simulink model "verify_Cooling_Tower_mdl"  (R2018b)
settings: Solver=ode45  StartTime=0  StopTime=1200  MaxStep=60  RelTol=1e-3  EnableMultiTasking=on
libraries: carnot x3
settings Model: Creator=drhf  LastModifiedBy=drhf
settings DataIOCC: SaveFormat=Array  SignalLoggingSaveFormat=ModelDataLogs
settings OptimizationCC: ExpressionDepthLimit=2147483647  LifeSpan=inf
settings DebuggingCC: UnderspecifiedInitializationDetection=Classic  MergeDetectMultiDrivingBlocksExec=none  SolverPrmCheckMsg=warning  FcnCallInpInsideContextMsg=warning  StateNameClashWarn=warning  SFUnexpectedBacktrackingDiag=warning  SFNoUnconditionalDefaultTransitionDiag=warning  SFExecutionAtInitializationDiag=none
settings HardwareCC: ProdBitPerPointer=32  ProdBitPerSizeT=32  ProdBitPerPtrDiffT=32  ProdLargestAtomicFloat=None  ProdIntDivRoundTo=Undefined  ProdEndianess=Unspecified  ProdWordSize=32  ProdHWDeviceType=32-bit Generic
settings ModelReferenceCC: PropagateSignalLabelsOutOfModel=off
settings SFSimCC: SimUseLocalCustomCode=off
settings RTWCC: RTWUseLocalCustomCode=off
settings CodeAppCC: StateflowObjectComments=on
settings GRTTargetCC: TargetLangStandard=C89/C90 (ANSI)  GeneratePreprocessorConditionals=Disable all  CombineOutputUpdateFcns=off  GRTInterface=on
settings ConfigComp: CovMetricSettings=dw  CovHtmlReporting=on  CovSaveCumulativeToWorkspaceVar=on  CovSaveSingleToWorkspaceVar=on  CovExternalEMLEnable=off

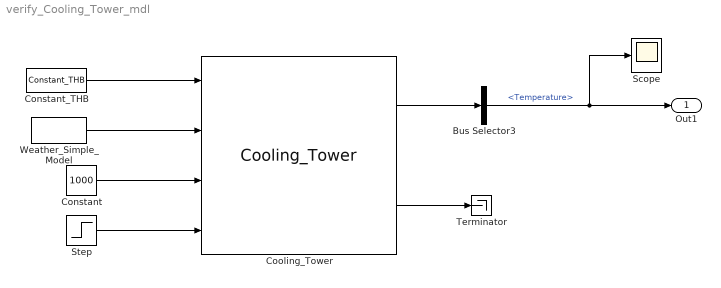
== system verify_Cooling_Tower_mdl ==
  Bus Selector3 : BusSelector  OutputSignals=Temperature
  Constant : Constant  Value=1000
  Constant_THB : carnot/Source/Simple/Constant_THB  t=15  mdot=1200/3600  p=1e5  mID=No Pressure Drop  fluid=Water  mix=0  mix2=0  mix3=0  dia=0.02  hgt=0
      settings: SourceProductName=Carnot
  Cooling_Tower : carnot/Source/Chiller/Cooling_Tower
      settings: SourceProductName=Carnot
  Scope : Scope
  Step : Step  Time=200  SampleTime=0
  Terminator : Terminator
  Weather_Simple_Model : carnot/Weather/Weather_Simple_Model  Ibn=900  Idg=100  tamb=5  deltaTsky=-6  rh=50  precip="10e-3/24/3600           % 10 mm in 24 h"  cloud=0.125  p=1013e2  vw=1  wdir=270  lat=60  colangle=0  colazi=0  colrot=0
      settings: SourceProductName=Carnot
  Out1 : Outport
  wires:
  Bus Selector3/1 -> Out1/1, Scope/1  "<Temperature>"
  Constant_THB/1 -> Cooling_Tower/1
  Step/1 -> Cooling_Tower/4
  Constant/1 -> Cooling_Tower/3
  Cooling_Tower/1 -> Bus Selector3/1
  Weather_Simple_Model/1 -> Cooling_Tower/2
  Cooling_Tower/2 -> Terminator/1
